simulink model "last_pressed_led_detectchange_fixed"  (R2025a)
settings: Solver=FixedStepDiscrete  StartTime=0.0  StopTime=20  FixedStep=1  RelTol=1e-3
libraries: simulink x2
settings Model: Creator=mahij  LastModifiedBy=mahij

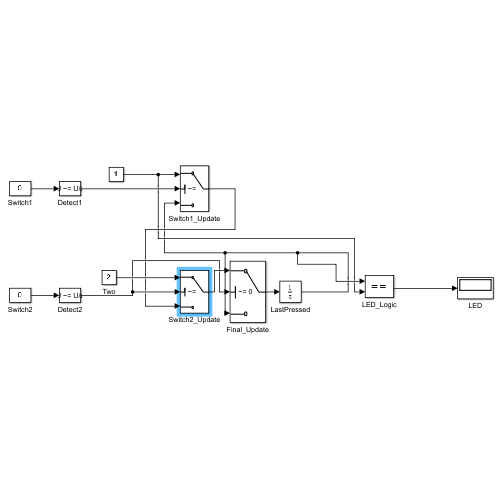
[thumbnail: Simulink's stored preview of the top-level diagram]
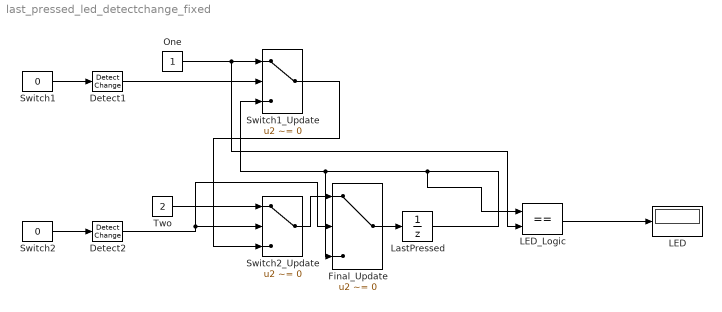
== system last_pressed_led_detectchange_fixed ==
  Detect1 : simulink/Logic and Bit Operations/Detect Change  vinit=0  OutDataTypeStr=boolean
  Detect2 : simulink/Logic and Bit Operations/Detect Change  vinit=0  OutDataTypeStr=boolean
  Final_Update : Switch  Criteria=u2 ~= 0  Threshold=0.5  SaturateOnIntegerOverflow=off  InputSameDT=off
  LED : Display
  LED_Logic : RelationalOperator  Operator===  OutDataTypeStr=boolean  RndMeth=Simplest  InputSameDT=off
  LastPressed : UnitDelay  HasFrameUpgradeWarning=on
  One : Constant
  Switch1 : Constant  Value=0
  Switch1_Update : Switch  Criteria=u2 ~= 0  Threshold=0.5  SaturateOnIntegerOverflow=off  InputSameDT=off
  Switch2 : Constant  Value=0
  Switch2_Update : Switch  Criteria=u2 ~= 0  Threshold=0.5  SaturateOnIntegerOverflow=off  InputSameDT=off
  Two : Constant  Value=2
  wires:
  Switch1/1 -> Detect1/1
  Switch2/1 -> Detect2/1
  One/1 -> LED_Logic/2, Switch1_Update/1
  Detect1/1 -> Switch1_Update/2
  LastPressed/1 -> Switch1_Update/3, Final_Update/3, LED_Logic/1
  Two/1 -> Switch2_Update/1
  Detect2/1 -> Switch2_Update/2, Final_Update/2
  Switch1_Update/1 -> Switch2_Update/3
  Switch2_Update/1 -> Final_Update/1
  Final_Update/1 -> LastPressed/1
  LED_Logic/1 -> LED/1
